simulink model "referee_update_handler"  (R2018a)
settings: Solver=VariableStepAuto  StartTime=0.0  StopTime=10.0  RelTol=1e-3
settings Model: Creator=blond  LastModifiedBy=blond

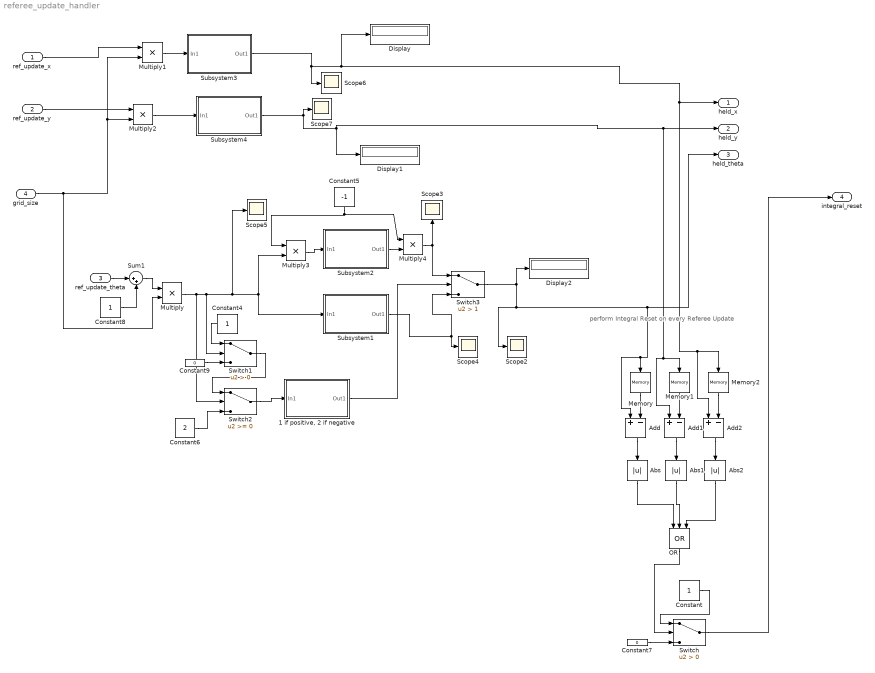
== system referee_update_handler ==
  note: perform
      | Integral
      | Reset on
      | every
      | Referee
      | Update
  ref_update_x : Inport
  ref_update_y : Inport  Port=2
  ref_update_theta : Inport  Port=3
  "grid_size " : Inport  Port=4
  "1 if positive, 2 if negative" : Subsystem
  Abs : Abs
  Abs1 : Abs
  Abs2 : Abs
  Add : Sum  Inputs=+-
  Add1 : Sum  Inputs=+-
  Add2 : Sum  Inputs=+-
  Constant : Constant
  Constant4 : Constant
  Constant5 : Constant  Value=-1
  Constant6 : Constant  Value=2
  Constant7 : Constant  Value=0
  Constant8 : Constant
  Constant9 : Constant  Value=0
  Display : Display
  Display1 : Display
  Display2 : Display
  Memory : Memory
  Memory1 : Memory
  Memory2 : Memory
  Multiply{,1..4} (5 alike) : Product
  OR : Logic  Operator=OR  Inputs=3  IconShape=distinctive  AllPortsSameDT=off  OutDataTypeStr=boolean
  Scope{2..7} (6 alike) : Scope
  Subsystem1 : Subsystem
  Subsystem2 : Subsystem
  Subsystem3 : Subsystem
  Subsystem4 : Subsystem
  Sum1 : Sum  Inputs=|++
  Switch : Switch  Criteria=u2 > Threshold
  Switch1 : Switch  Criteria=u2 > Threshold
  Switch2 : Switch
  Switch3 : Switch  Criteria=u2 > Threshold  Threshold=1
  held_x : Outport
  held_y : Outport  Port=2
  held_theta : Outport  Port=3
  integral_reset : Outport  Port=4
  wires:
  Multiply/1 -> Switch2/2, Switch1/2, Multiply3/2, Subsystem1/1(In1), Scope5/1
  Constant6/1 -> Switch2/3
  Subsystem2/1(Out1) -> Multiply4/2
  Constant8/1 -> Sum1/2
  ref_update_x/1 -> Multiply1/1
  ref_update_y/1 -> Multiply2/1
  Add1/1 -> Abs1/1
  Subsystem1/1(Out1) -> Switch3/3, Scope4/1
  Constant7/1 -> Switch/3
  OR/1 -> Switch/2
  Subsystem3/1(Out1) -> Scope6/1, held_x/1, Memory2/1, Add2/1, Display/1
  Switch2/1 -> "1 if positive, 2 if negative"/1(In1)
  "1 if positive, 2 if negative"/1(Out1) -> Switch3/2
  Abs/1 -> OR/1
  ref_update_theta/1 -> Sum1/1
  Add2/1 -> Abs2/1
  Constant4/1 -> Switch1/1
  Multiply2/1 -> Subsystem4/1(In1)
  Constant/1 -> Switch/1
  Multiply1/1 -> Subsystem3/1(In1)
  Switch1/1 -> Switch2/1
  Constant5/1 -> Multiply4/1, Multiply3/1
  Switch/1 -> integral_reset/1
  Abs1/1 -> OR/2
  Constant9/1 -> Switch1/3
  Abs2/1 -> OR/3
  Multiply3/1 -> Subsystem2/1(In1)
  Switch3/1 -> Scope2/1, held_theta/1, Memory/1, Add/1, Display2/1
  Sum1/1 -> Multiply/1
  Subsystem4/1(Out1) -> held_y/1, Add1/1, Memory1/1, Display1/1, Scope7/1
  Add/1 -> Abs/1
  Memory/1 -> Add/2
  Memory2/1 -> Add2/2
  Multiply4/1 -> Scope3/1, Switch3/1
  "grid_size "/1 -> Multiply/2, Multiply1/2, Multiply2/2
  Memory1/1 -> Add1/2

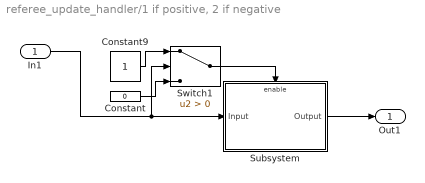
== system referee_update_handler/1 if positive, 2 if negative ==
  In1 : Inport
  Constant : Constant  Value=0
  Constant9 : Constant
  Subsystem : Subsystem
  Switch1 : Switch  Criteria=u2 > Threshold
  Out1 : Outport
  wires:
  Constant9/1 -> Switch1/1
  In1/1 -> Switch1/2, Subsystem/1(Input)
  Switch1/1 -> Subsystem/Enable
  Subsystem/1(Output) -> Out1/1
  Constant/1 -> Switch1/3

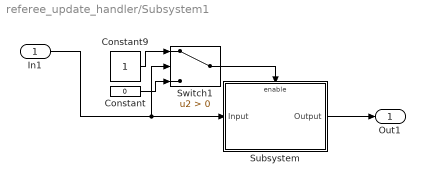
== system referee_update_handler/Subsystem1 ==
  In1 : Inport
  Constant : Constant  Value=0
  Constant9 : Constant
  Subsystem : Subsystem
  Switch1 : Switch  Criteria=u2 > Threshold
  Out1 : Outport
  wires:
  Constant9/1 -> Switch1/1
  In1/1 -> Switch1/2, Subsystem/1(Input)
  Switch1/1 -> Subsystem/Enable
  Subsystem/1(Output) -> Out1/1
  Constant/1 -> Switch1/3

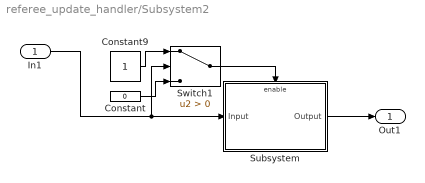
== system referee_update_handler/Subsystem2 ==
  In1 : Inport
  Constant : Constant  Value=0
  Constant9 : Constant
  Subsystem : Subsystem
  Switch1 : Switch  Criteria=u2 > Threshold
  Out1 : Outport
  wires:
  Constant9/1 -> Switch1/1
  In1/1 -> Switch1/2, Subsystem/1(Input)
  Switch1/1 -> Subsystem/Enable
  Subsystem/1(Output) -> Out1/1
  Constant/1 -> Switch1/3

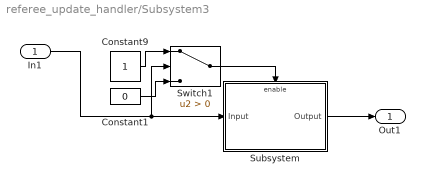
== system referee_update_handler/Subsystem3 ==
  In1 : Inport
  Constant1 : Constant  Value=0
  Constant9 : Constant
  Subsystem : Subsystem
  Switch1 : Switch  Criteria=u2 > Threshold
  Out1 : Outport
  wires:
  Constant9/1 -> Switch1/1
  In1/1 -> Switch1/2, Subsystem/1(Input)
  Switch1/1 -> Subsystem/Enable
  Subsystem/1(Output) -> Out1/1
  Constant1/1 -> Switch1/3

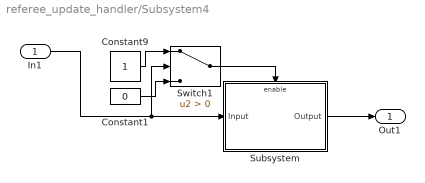
== system referee_update_handler/Subsystem4 ==
  In1 : Inport
  Constant1 : Constant  Value=0
  Constant9 : Constant
  Subsystem : Subsystem
  Switch1 : Switch  Criteria=u2 > Threshold
  Out1 : Outport
  wires:
  Constant9/1 -> Switch1/1
  In1/1 -> Switch1/2, Subsystem/1(Input)
  Switch1/1 -> Subsystem/Enable
  Subsystem/1(Output) -> Out1/1
  Constant1/1 -> Switch1/3

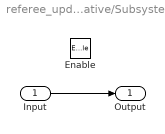
== system referee_update_handler/1 if positive, 2 if negative/Subsystem ==
  Input : Inport
  Enable : EnablePort
  Output : Outport
  wires:
  Input/1 -> Output/1

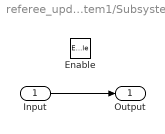
== system referee_update_handler/Subsystem1/Subsystem ==
  Input : Inport
  Enable : EnablePort
  Output : Outport
  wires:
  Input/1 -> Output/1

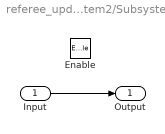
== system referee_update_handler/Subsystem2/Subsystem ==
  Input : Inport
  Enable : EnablePort
  Output : Outport
  wires:
  Input/1 -> Output/1

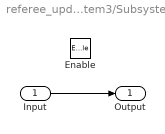
== system referee_update_handler/Subsystem3/Subsystem ==
  Input : Inport
  Enable : EnablePort
  Output : Outport
  wires:
  Input/1 -> Output/1

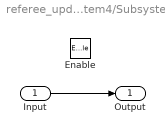
== system referee_update_handler/Subsystem4/Subsystem ==
  Input : Inport
  Enable : EnablePort
  Output : Outport
  wires:
  Input/1 -> Output/1
